simulink model "simulink1"  (R2017a)
settings: Solver=VariableStepAuto  StartTime=0.0  StopTime=4000.0  RelTol=1e-3
libraries: cstblocks x5
settings Model: Creator=Night_Fury  LastModifiedBy=Havoc

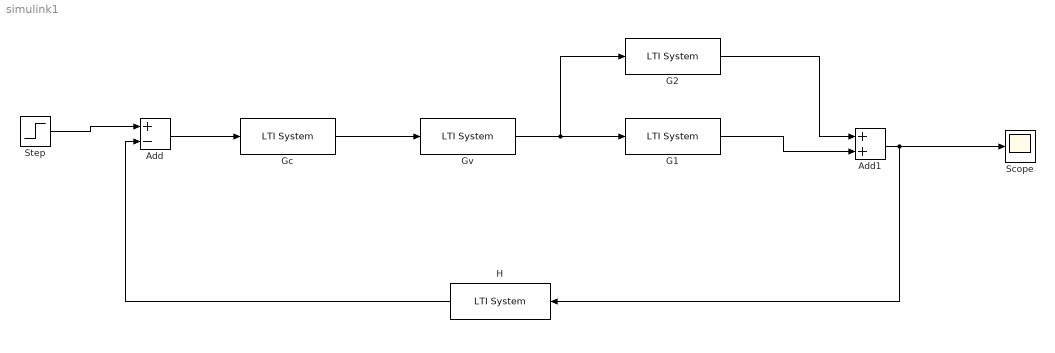
== system simulink1 ==
  Add : Sum  Inputs=+-
  Add1 : Sum
  G1 : cstblocks/LTI System  sys=tf(1,[1 1])  IC=[]
  G2 : cstblocks/LTI System  sys=tf(1,[1 1 8])  IC=[]
  Gc : cstblocks/LTI System  sys=tf(10,[2 1])  IC=[]
  Gv : cstblocks/LTI System  sys="tf(20,[1  1])"  IC=[]
  H : cstblocks/LTI System  sys=tf(5 ,[ 1 0])  IC=[]
  Scope : Scope
  Step : Step  SampleTime=0
  wires:
  Step/1 -> Add/1
  Add/1 -> Gc/1
  Gc/1 -> Gv/1
  Gv/1 -> G2/1, G1/1
  G1/1 -> Add1/2
  G2/1 -> Add1/1
  Add1/1 -> Scope/1, H/1
  H/1 -> Add/2
